simulink model "PID_Regulation"  (R2020a)
settings: Solver=ode3  StartTime=0.0  StopTime=inf  RelTol=1e-3  EnableMultiTasking=on
libraries: arduinolib x4
settings Model: FPTRunName=Active  SILPILModeSetting=veronly  ExtModeTrigDuration=2  Creator=The MathWorks, Inc.  LastModifiedBy=vince
settings DataIOCC: LimitDataPoints=on  SaveFormat=Array  ReturnWorkspaceOutputs=off
settings OptimizationCC: ExpressionDepthLimit=2147483647  LifeSpan=Inf  MaxStackSize=64
settings DebuggingCC: UnderspecifiedInitializationDetection=Classic  MergeDetectMultiDrivingBlocksExec=none  FcnCallInpInsideContextMsg=warning  AllowSymbolicDim=off  StateNameClashWarn=warning  SFUnexpectedBacktrackingDiag=warning  SFNoUnconditionalDefaultTransitionDiag=warning  SFExecutionAtInitializationDiag=none  ArithmeticOperatorsInVariantConditions=warning
settings HardwareCC: ProdBitPerInt=16  ProdBitPerPointer=16  ProdBitPerSizeT=16  ProdBitPerPtrDiffT=16  ProdLargestAtomicFloat=None  ProdWordSize=8  ProdHWDeviceType=Atmel->AVR
settings ModelReferenceCC: PropagateSignalLabelsOutOfModel=off
settings SFSimCC: SimUseLocalCustomCode=off  MATLABDynamicMemAlloc=off
settings RTWCC: SystemTargetFile=ert.tlc  HardwareBoard=Arduino Uno  TemplateMakefile=ert_default_tmf  GenerateReport=on  RTWVerbose=off  RTWUseLocalCustomCode=off  Toolchain=Arduino AVR  BuildConfiguration=Faster Runs  LaunchReport=on
settings CodeAppCC: ForceParamTrailComments=on  OperatorAnnotations=on  StateflowObjectComments=on  MATLABSourceComments=on
settings ERTTargetCC: MultiwordLength=2048  ERTCustomFileBanners=off  SupportContinuousTime=on  SupportNonInlinedSFcns=on  RemoveResetFunc=off  SupportVariableSizeSignals=on  ModelStepFunctionPrototypeControlCompliant=off  ExtModeStaticAllocSize=250
settings ConfigComp: CovMetricSettings=dw  CovHtmlReporting=on  CovSaveCumulativeToWorkspaceVar=on  CovSaveSingleToWorkspaceVar=on  CovExternalEMLEnable=off  CovSFcnEnable=off

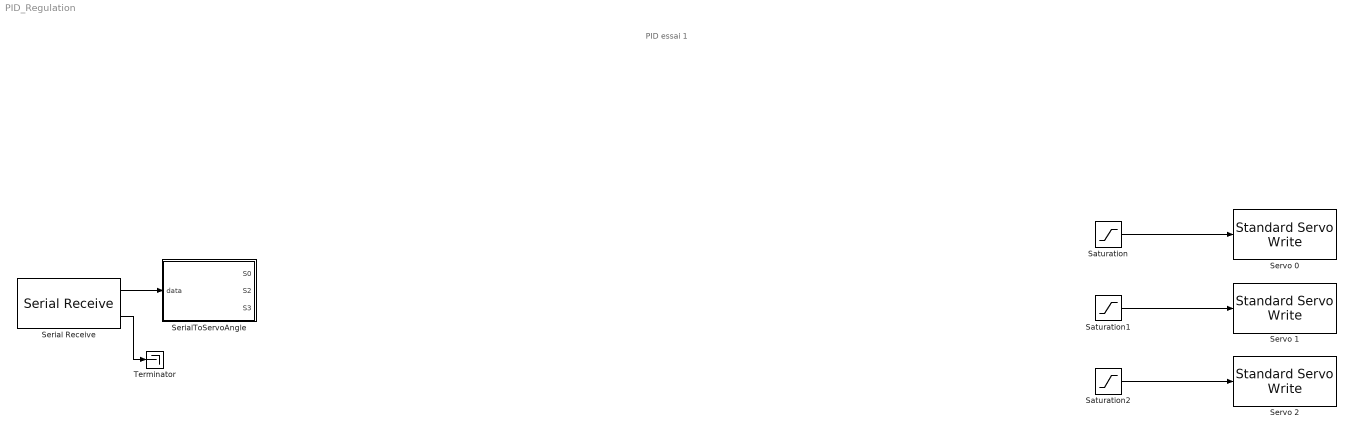
== system PID_Regulation ==
  note: PID essai 1
  Saturation : Saturate  UpperLimit=60  LowerLimit=0
  Saturation1 : Saturate  UpperLimit=60  LowerLimit=0
  Saturation2 : Saturate  UpperLimit=60  LowerLimit=0
  Serial Receive : arduinolib/Serial Receive  isARMArch=off  portNumber=0  DataType=int32  Datalength=[2]  SampleTime=0.1  showOutStatus=on  blockPlatform=arduino
      settings: SourceProductBaseCode=ARDUINO
  SerialToServoAngle : MATLAB Function  TreatAsAtomicUnit=on
  Servo 0 : arduinolib/Standard Servo Write  pinNumber=3  ServoIndex=0  blockPlatform=ARDUINO
  Servo 1 : arduinolib/Standard Servo Write  pinNumber=5  ServoIndex=1  blockPlatform=ARDUINO
  Servo 2 : arduinolib/Standard Servo Write  pinNumber=6  ServoIndex=2  blockPlatform=ARDUINO
  Terminator : Terminator
  wires:
  Saturation/1 -> Servo 0/1
  Saturation2/1 -> Servo 2/1
  Saturation1/1 -> Servo 1/1
  Serial Receive/2 -> Terminator/1
  Serial Receive/1 -> SerialToServoAngle/1(data)
  ? -> Saturation1/1
  ? -> Saturation/1
  ? -> Saturation2/1

== matlab function PID_Regulation/SerialToServoAngle ==
  data: S0 output; data input; S2 output; S3 output
function [S0,S2, S3] = SerialToCoordinates(data)
S0=int32(data(1));
S2=int32(data(2));
S3=int32(data(3));
